simulink model "test"  (R2018b)
settings: Solver=ode4  StartTime=0.0  StopTime=15  FixedStep=0.03  RelTol=1e-3
values from neighbouring files (symbols this model uses):
  h = 5000    [test.m]
  tt = 15    [test.m]
settings Model: Creator=ysq  LastModifiedBy=ysq

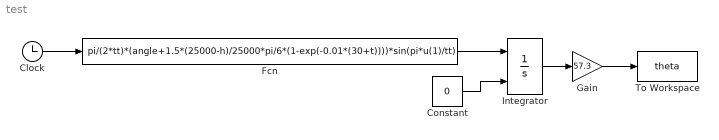
== system test ==
  Clock : Clock
  Constant : Constant  Value=0
  Fcn : Fcn  Expr=pi/(2*tt)*(angle+1.5*(25000-h)/25000*pi/6*(1-exp(-0.01*(30+t))))*sin(pi*u(1)/tt)
  Gain : Gain  Gain=57.3
  Integrator : Integrator  InitialConditionSource=external
  To Workspace : ToWorkspace  VariableName=theta  SampleTime=-1
  wires:
  Clock/1 -> Fcn/1
  Fcn/1 -> Integrator/1
  Constant/1 -> Integrator/2
  Integrator/1 -> Gain/1
  Gain/1 -> To Workspace/1
